simulink model "PUSlab6sim"  (R2022b)
settings: Solver=VariableStepAuto  StartTime=0.0  StopTime=czas_systemu  RelTol=1e-3
values from neighbouring files (symbols this model uses):
  Cvp = cp*rop*Vp    (= 33600)    [PUSlab6v2.m]
  Cvw = cp*rop*Vw    (= 67200)    [PUSlab6v2.m]
  dqg = 0.1*q_g_N    (= 1000)    [PUSlab6v2.m]
  dTzew = 0    [PUSlab6v2.m]
  K_cp = ((a1*q_g_N)*(T_wew_N-Tp_N))/((Tp_N-T_zew_N)*(T_wew_N-T_zew_N+a1*(T_wew_N-Tp_N)))    (= 23.2558139535)    [PUSlab6v2.m]
  K_cw = (q_g_N)/(T_wew_N-T_zew_N+a1*(T_wew_N-Tp_N))    (= 232.558139535)    [PUSlab6v2.m]
  K_cwp = (a1*(q_g_N))/(T_wew_N-T_zew_N+a1*(T_wew_N-Tp_N))    (= 69.7674418605)    [PUSlab6v2.m]
  Kp = 3.15    [PUSlab6v2.m]
  L11 = [ksTwew]    [PUSlab6v2.m]
  L12 = [ksTp]    [PUSlab6v2.m]
  L21 = [kmdTwew]    [PUSlab6v2.m]
  L22 = [kmdTp]    [PUSlab6v2.m]
  M1 = [T,1]    [PUSlab6v2.m]
  M2 = [T_sp,1]    [PUSlab6v2.m]
  M3 = [T2,1]    [PUSlab6v2.m]
  M4 = [T3,1]    [PUSlab6v2.m]
  q_g_0 = q_g_N    (= 10000)    [PUSlab6v2.m]
  t0 = 1000    [PUSlab6v2.m]
  T_0_tp = 100    [PUSlab6v2.m]
  T_0_wew = 0    [PUSlab6v2.m]
  T_wew_0 = (q_g_0+K_cw*T_zew_0+a1*K_cw*Tp_0)/(K_cw+K_cwp)    (= 20)    [PUSlab6v2.m]
  T_zew_0 = T_zew_N    (= -20)    [PUSlab6v2.m]
  Td = 50    [PUSlab6v2.m]
  Ti = 333    [PUSlab6v2.m]
  To = t_2w-T2    (= 0)    [PUSlab6v2.m]
  To1 = t_2p-T3    (= 175)    [PUSlab6v2.m]
  Tp_0 = (K_cp*T_zew_0*(K_cw+K_cwp)+K_cwp*(q_g_0+K_cw*T_zew_0))/(K_cw*K_cwp+K_cw*K_cp+K_cwp*K_cp)    (= 10)    [PUSlab6v2.m]
settings Model: Creator=Mariusz  LastModifiedBy=Dawid
settings DataIOCC: ReturnWorkspaceOutputs=off
settings DebuggingCC: UnconnectedInputMsg=warning  UnconnectedOutputMsg=warning  UnconnectedLineMsg=warning
settings ModelReferenceCC: EnableRefExpFcnMdlSchedulingChecks=on
settings RTWCC: DLArmComputeVersion=19.05

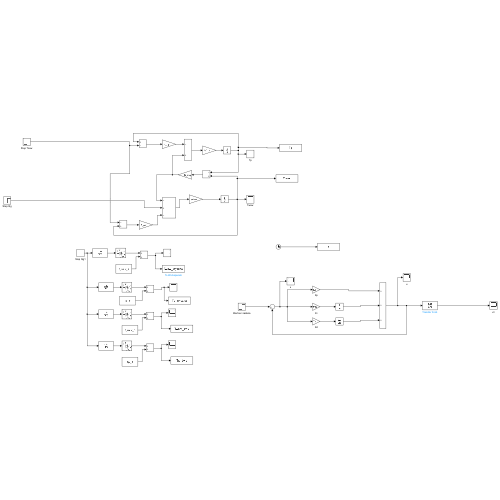
[thumbnail: Simulink's stored preview of the top-level diagram]
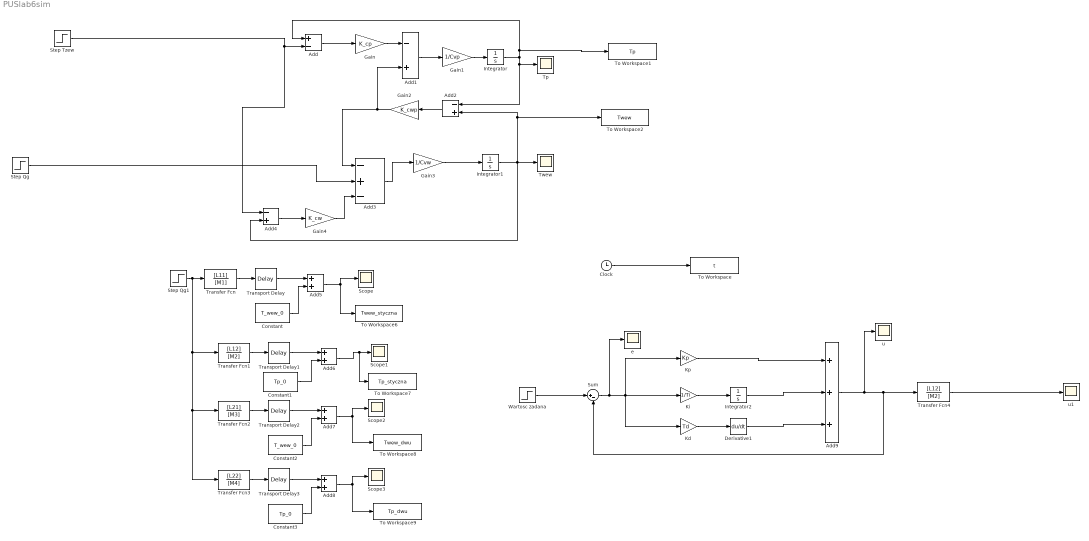
== system PUSlab6sim ==
  Add : Sum  Inputs=+-
  Add1 : Sum  Inputs=-+
  Add2 : Sum  Inputs=-+
  Add3 : Sum  Inputs=-+-
  Add4 : Sum  Inputs=-+
  Add{5..8} (4 alike) : Sum
  Add9 : Sum  Inputs=+++
  Clock : Clock
  Constant : Constant  Value=T_wew_0
  Constant1 : Constant  Value=Tp_0
  Constant2 : Constant  Value=T_wew_0
  Constant3 : Constant  Value=Tp_0
  Derivative1 : Derivative
  Gain : Gain  Gain=K_cp
  Gain1 : Gain  Gain=1/Cvp
  Gain2 : Gain  Gain=K_cwp
  Gain3 : Gain  Gain=1/Cvw
  Gain4 : Gain  Gain=K_cw
  Integrator : Integrator  InitialCondition=Tp_0
  Integrator1 : Integrator  InitialCondition=T_wew_0
  Integrator2 : Integrator  InitialCondition=q_g_0
  Kd : Gain  Gain=Td
  Ki : Gain  Gain=1/Ti
  Kp : Gain  Gain=Kp
  Scope{,1..3} (4 alike) : Scope
  Step Qg : Step  Time=t0  Before=q_g_0  After=q_g_0+dqg  SampleTime=0
  Step Qg1 : Step  Time=t0  After=dqg  SampleTime=0
  Step Tzew : Step  Time=t0  Before=T_zew_0  After=T_zew_0+dTzew  SampleTime=0
  Sum : Sum  Inputs=|+-
  To Workspace : ToWorkspace  VariableName=t  SaveFormat=Timeseries  SampleTime=-1
  To Workspace1 : ToWorkspace  VariableName=Tp  SampleTime=-1
  To Workspace2 : ToWorkspace  VariableName=Twew  SampleTime=-1
  To Workspace6 : ToWorkspace  VariableName=Twew_styczna  SampleTime=-1
  To Workspace7 : ToWorkspace  VariableName=Tp_styczna  SampleTime=-1
  To Workspace8 : ToWorkspace  VariableName=Twew_dwu  SampleTime=-1
  To Workspace9 : ToWorkspace  VariableName=Tp_dwu  SampleTime=-1
  Tp : Scope
  Transfer Fcn : TransferFcn  Numerator=[L11]  Denominator=[M1]
  Transfer Fcn1 : TransferFcn  Numerator=[L12]  Denominator=[M2]
  Transfer Fcn2 : TransferFcn  Numerator=[L21]  Denominator=[M3]
  Transfer Fcn3 : TransferFcn  Numerator=[L22]  Denominator=[M4]
  Transfer Fcn4 : TransferFcn  Numerator=[L12]  Denominator=[M2]
  Transport Delay : TransportDelay  DelayTime=T_0_wew
  Transport Delay1 : TransportDelay  DelayTime=T_0_tp
  Transport Delay2 : TransportDelay  DelayTime=To
  Transport Delay3 : TransportDelay  DelayTime=To1
  Twew : Scope
  Wartosc zadana : Step  Time=t0  Before=10  After=15  SampleTime=0
  e : Scope
  u : Scope
  u1 : Scope
  wires:
  Clock/1 -> To Workspace/1
  Step Tzew/1 -> Add4/1, Add/2
  Add/1 -> Gain/1
  Gain/1 -> Add1/1
  Add1/1 -> Gain1/1
  Gain1/1 -> Integrator/1
  Integrator/1 -> Add2/1, Tp/1, To Workspace1/1, Add/1
  Add2/1 -> Gain2/1
  Gain2/1 -> Add3/1, Add1/2
  Integrator1/1 -> Add4/2, Twew/1, To Workspace2/1, Add2/2
  Step Qg/1 -> Add3/2
  Gain3/1 -> Integrator1/1
  Add3/1 -> Gain3/1
  Gain4/1 -> Add3/3
  Add4/1 -> Gain4/1
  Transfer Fcn/1 -> Transport Delay/1
  Transport Delay/1 -> Add5/1
  Add5/1 -> Scope/1, To Workspace6/1
  Constant/1 -> Add5/2
  Transport Delay1/1 -> Add6/1
  Constant1/1 -> Add6/2
  Add6/1 -> To Workspace7/1, Scope1/1
  Transfer Fcn1/1 -> Transport Delay1/1
  Transport Delay2/1 -> Add7/1
  Constant2/1 -> Add7/2
  Add7/1 -> Scope2/1, To Workspace8/1
  Transfer Fcn2/1 -> Transport Delay2/1
  Step Qg1/1 -> Transfer Fcn1/1, Transfer Fcn3/1, Transfer Fcn2/1, Transfer Fcn/1
  Add8/1 -> To Workspace9/1, Scope3/1
  Transfer Fcn3/1 -> Transport Delay3/1
  Transport Delay3/1 -> Add8/1
  Constant3/1 -> Add8/2
  Derivative1/1 -> Add9/3
  Integrator2/1 -> Add9/2
  Kd/1 -> Derivative1/1
  Kp/1 -> Add9/1
  Sum/1 -> e/1, Ki/1, Kp/1, Kd/1
  Ki/1 -> Integrator2/1
  Wartosc zadana/1 -> Sum/1
  Add9/1 -> u/1, Sum/2, Transfer Fcn4/1
  Transfer Fcn4/1 -> u1/1
